simulink subsystem "DLBattery"  (R2025b)
settings: Solver=VariableStepAuto  StartTime=0.0  StopTime=10.0  RelTol=1e-3
undefined symbols (not defined in the file): BattAmpHr, BattCurr, BattPwr, BattPwrLoss, BattSoc, BattTemp, BattVolt, PlntBattNumCellSer, PlntDLBatt_CellNomVolt, PlntDLBatt_InitialTemp, PlntDLBatt_muOutput, PlntDLBatt_sigInput, PlntDLBatt_sigOutput, PlntDLBattCapInit, PlntDLBattChrgMax, PlntDLBattNumCellPar, PlntDLBattNumCellSer
libraries: slident x1
settings Model: ModifiedByFormat=The MathWorks, Inc.  Creator=The MathWorks, Inc.  LastModifiedBy=The MathWorks, Inc.
settings SolverCC: MaxZcPerStep=1.0
settings OptimizationCC: ReuseModelBlockBuffer=off
settings DebuggingCC: UnconnectedInputMsg=warning  UnconnectedOutputMsg=warning  UnconnectedLineMsg=warning  SubsystemReferenceDiagnosticForUnitTest=warning
settings ModelReferenceCC: EnableRefExpFcnMdlSchedulingChecks=on
settings RTWCC: GPUComputeCapability=3.5  DLArmComputeVersion=19.05

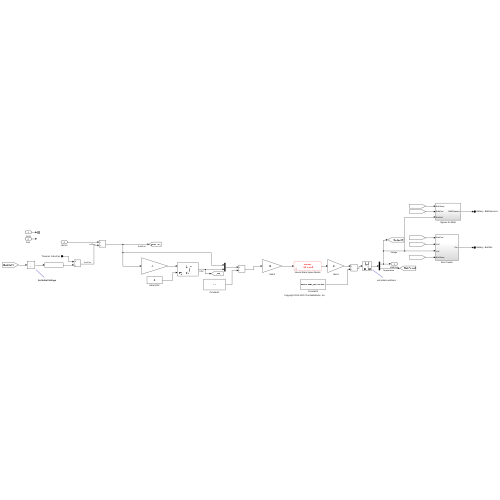
[thumbnail: Simulink's stored preview of the top-level diagram]
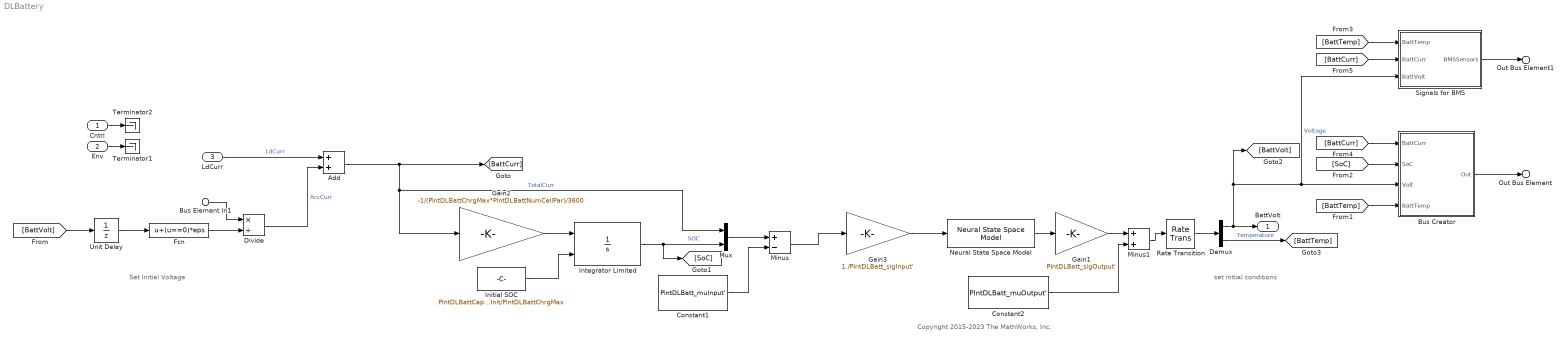
== system DLBattery ==
  note: set initial conditions
  note: Set Initial Voltage
  note: Copyright 2015-2023 The MathWorks, Inc.
  Cntrl : Inport
  Env : Inport  Port=2
  LdCurr : Inport  Port=3
  Bus Element In1 : Inport  Port=4  PortName=Thermal  Element=EAccPwr
  Add : Sum
  Bus Creator : Subsystem
  Constant1 : Constant  Value=PlntDLBatt_muInput'
  Constant2 : Constant  Value=PlntDLBatt_muOutput'
  Demux : Demux  Outputs=2
  Divide : Product  Inputs=*/
  Fcn : Fcn  Expr=u+(u==0)*eps
  Gain1 : Gain  Gain=PlntDLBatt_sigOutput'
  Gain2 : Gain  Gain=-1/(PlntDLBattChrgMax*PlntDLBattNumCellPar)/3600
  Gain3 : Gain  Gain=1./PlntDLBatt_sigInput'
  Initial SOC : Constant  Value=PlntDLBattCapInit/PlntDLBattChrgMax
  Integrator Limited : Integrator  InitialConditionSource=external  LimitOutput=on  UpperSaturationLimit=1  LowerSaturationLimit=0
  Minus : Sum  Inputs=+-
  Minus1 : Sum
  Mux : Mux  Inputs=2
  Neural State Space Model : slident/Models/Neural State Space Model  sys=PlntDLBattNeuralODE.NeuralSSObj  x0type=internal  ic=([PlntDLBatt_CellNomVolt*PlntDLBattNumCellSer PlntDLBatt_InitialTemp]-PlntDLBatt_muOutput)./PlntDLBatt_sigOutput  returnx=off  returndx=off  domain=DT  feedthroughCT=NoFT  feedthroughDT=NoFT
  Rate Transition : RateTransition  InitialCondition=[PlntDLBatt_CellNomVolt PlntDLBatt_InitialTemp]  OutPortSampleTime=0.1
  Signals for BMS : Subsystem
  Terminator1 : Terminator
  Terminator2 : Terminator
  Unit Delay : UnitDelay  InitialCondition=PlntDLBatt_CellNomVolt*PlntBattNumCellSer  SampleTime=-1  HasFrameUpgradeWarning=on
  BattVolt : Outport  VectorParamsAs1DForOutWhenUnconnected=off
  Out Bus Element : Outport  Port=2  PortName=Battery  Element=BattInfo
  Out Bus Element1 : Outport  Port=2  PortName=Battery  Element=BMSSensors
  wires:
  Divide/1 -> Add/2  "AccCurr"
  Demux/1 -> BattVolt/1, Signals for BMS/3(BattVolt), Bus Creator/3(Volt), [BattVolt]  "Voltage"
  LdCurr/1 -> Add/1  "LdCurr"
  [BattTemp] -> Signals for BMS/1(BattTemp)
  Bus Creator/1(Out) -> Out Bus Element/1
  Signals for BMS/1(BMSSensors) -> Out Bus Element1/1
  Demux/2 -> [BattTemp]  "Temperature"
  [BattTemp] -> Bus Creator/4(BattTemp)
  Fcn/1 -> Divide/2
  Bus Element In1/1 -> Divide/1
  Gain3/1 -> Neural State Space Model/1
  Neural State Space Model/1 -> Gain1/1
  Constant1/1 -> Minus/2
  Minus/1 -> Gain3/1
  Initial SOC/1 -> Integrator Limited/2
  Integrator Limited/1 -> [SoC], Mux/2  "SOC"
  Gain2/1 -> Integrator Limited/1
  Mux/1 -> Minus/1
  Gain1/1 -> Minus1/1
  Rate Transition/1 -> Demux/1
  [BattCurr] -> Bus Creator/1(BattCurr)
  [SoC] -> Bus Creator/2(SoC)
  [BattCurr] -> Signals for BMS/2(BattCurr)
  [BattVolt] -> Unit Delay/1
  Unit Delay/1 -> Fcn/1
  Env/1 -> Terminator1/1
  Cntrl/1 -> Terminator2/1
  Add/1 -> Gain2/1, Mux/1, [BattCurr]  "TotalCurr"
  Constant2/1 -> Minus1/2
  Minus1/1 -> Rate Transition/1

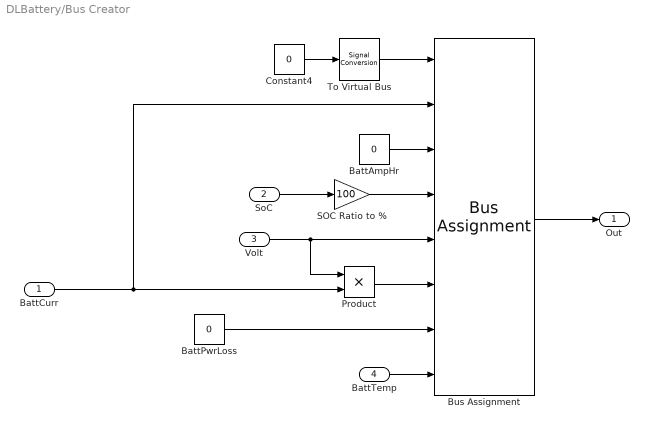
== system DLBattery/Bus Creator ==
  BattCurr : Inport
  SoC : Inport  Port=2
  Volt : Inport  Port=3
  BattTemp : Inport  Port=4
  BattAmpHr : Constant  Value=0
  BattPwrLoss : Constant  Value=0
  Bus Assignment : BusAssignment  AssignedSignals=BattCurr,BattAmpHr,BattSoc,BattVolt,BattPwr,BattPwrLoss,BattTemp
  Constant4 : Constant  Value=0  OutDataTypeStr=Bus: BattInfo  SampleTime=Inf
  Product : Product
  SOC Ratio to % : Gain  Gain=100
  To Virtual Bus : SignalConversion  ConversionOutput=Virtual bus  OverrideOpt=off
  Out : Outport
  wires:
  BattTemp/1 -> Bus Assignment/8
  Bus Assignment/1 -> Out/1
  Product/1 -> Bus Assignment/6
  BattPwrLoss/1 -> Bus Assignment/7
  SoC/1 -> SOC Ratio to %/1
  Constant4/1 -> To Virtual Bus/1
  To Virtual Bus/1 -> Bus Assignment/1
  Volt/1 -> Bus Assignment/5, Product/1
  SOC Ratio to %/1 -> Bus Assignment/4
  BattCurr/1 -> Bus Assignment/2, Product/2
  BattAmpHr/1 -> Bus Assignment/3

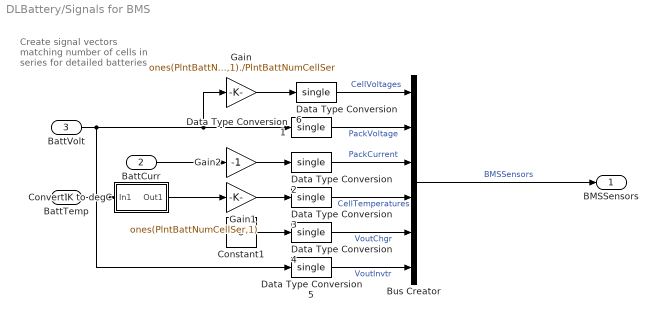
== system DLBattery/Signals for BMS ==
  note: Create signal vectors
      | matching number of
      | cells in series for
      | detailed batteries
  BattTemp : Inport
  BattCurr : Inport  Port=2
  BattVolt : Inport  Port=3
  Bus Creator : BusCreator  Inputs=6
  Constant1 : Constant  Value=0
  Convert K to degC : Subsystem
  Data Type Conversion{1..6} (6 alike) : DataTypeConversion  OutDataTypeStr=single  SaturateOnIntegerOverflow=off  RndMeth=Floor
  Gain : Gain  Gain=ones(PlntBattNumCellSer,1)./PlntBattNumCellSer
  Gain1 : Gain  Gain=ones(PlntBattNumCellSer,1)
  Gain2 : Gain  Gain=-1
  BMSSensors : Outport
  wires:
  BattCurr/1 -> Gain2/1
  Constant1/1 -> Data Type Conversion4/1
  BattVolt/1 -> Data Type Conversion1/1, Gain/1, Data Type Conversion5/1
  Gain/1 -> Data Type Conversion6/1
  BattTemp/1 -> Convert K to degC/1(In1)
  Data Type Conversion4/1 -> Bus Creator/5  "VoutChgr"
  Gain1/1 -> Data Type Conversion3/1
  Data Type Conversion5/1 -> Bus Creator/6  "VoutInvtr"
  Gain2/1 -> Data Type Conversion2/1
  Convert K to degC/1(Out1) -> Gain1/1
  Data Type Conversion1/1 -> Bus Creator/2  "PackVoltage"
  Data Type Conversion6/1 -> Bus Creator/1  "CellVoltages"
  Data Type Conversion2/1 -> Bus Creator/3  "PackCurrent"
  Data Type Conversion3/1 -> Bus Creator/4  "CellTemperatures"
  Bus Creator/1 -> BMSSensors/1  "BMSSensors"

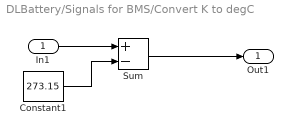
== system DLBattery/Signals for BMS/Convert K to degC ==
  In1 : Inport
  Constant1 : Constant  Value=273.15
  Sum : Sum  Inputs=+-
  Out1 : Outport
  wires:
  Sum/1 -> Out1/1
  Constant1/1 -> Sum/2
  In1/1 -> Sum/1
